simulink subsystem "Drive_Motor"  (R2025b)
settings: Solver=VariableStepAuto  StartTime=0.0  StopTime=10.0  RelTol=1e-3
model mask{channel=0}
  mask prompts: channel "Servo Channel (0-15)"
libraries: raspberrypiCommlib x5
settings Model: Creator=Maken  LastModifiedBy=Maken

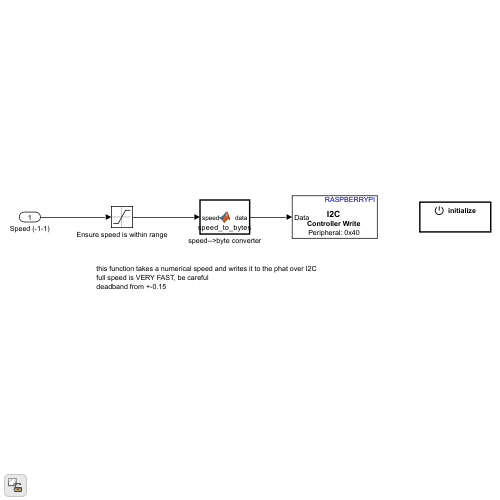
[thumbnail: Simulink's stored preview of the top-level diagram]
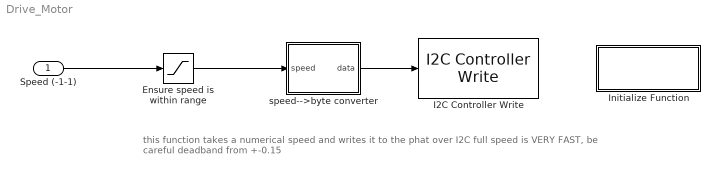
== system Drive_Motor ==
  note: this function takes a numerical speed and writes it to the phat over I2C
      | full speed is VERY FAST, be careful
      | deadband from +-0.15
  Speed (-1-1) : Inport
  Ensure speed is within range : Saturate  UpperLimit=1  LowerLimit=-1
  I2C Controller Write : raspberrypiCommlib/I2C Controller Write  BoardProperty=Pi 5 Model  I2CModule=1  Mode=Master  SlaveAddress=0x40  SlaveByteOrder=LittleEndian  Direction=Transmitter  RegisterAddressMode=on  RegisterAddress=0x06 + (channel * 4)  SlaveDataType=uint8  DataLength=1  NoAck=off  RepeatedStart=off  OutputStatus=off
  Initialize Function : Subsystem  TreatAsAtomicUnit=on
  speed-->byte converter : MATLAB Function  TreatAsAtomicUnit=on
  wires:
  Speed (-1-1)/1 -> Ensure speed is within range/1
  Ensure speed is within range/1 -> speed-->byte converter/1(speed)
  speed-->byte converter/1(data) -> I2C Controller Write/1

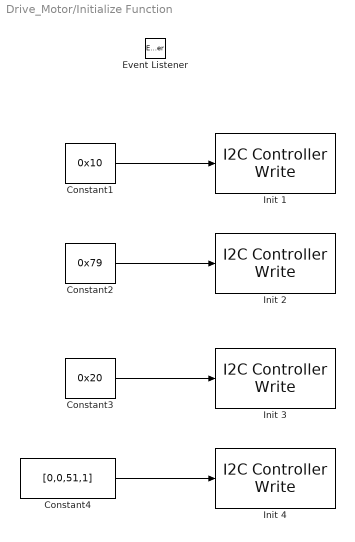
== system Drive_Motor/Initialize Function ==
  Constant1 : Constant  Value=0x10
  Constant2 : Constant  Value=0x79
  Constant3 : Constant  Value=0x20
  Constant4 : Constant  Value=[0,0,51,1]  OutDataTypeStr=uint8
  Event Listener : EventListener  DisableCoverage=on  EventName=reset
  Init 1 : raspberrypiCommlib/I2C Controller Write  BoardProperty=Pi 5 Model  I2CModule=1  Mode=Master  SlaveAddress=0x40  SlaveByteOrder=LittleEndian  Direction=Transmitter  RegisterAddressMode=on  RegisterAddress=0x00  SlaveDataType=uint8  DataLength=1  NoAck=off  RepeatedStart=off  OutputStatus=off
  Init 2 : raspberrypiCommlib/I2C Controller Write  BoardProperty=Pi 5 Model  I2CModule=1  Mode=Master  SlaveAddress=0x40  SlaveByteOrder=LittleEndian  Direction=Transmitter  RegisterAddressMode=on  RegisterAddress=0xFE  SlaveDataType=uint8  DataLength=1  NoAck=off  RepeatedStart=off  OutputStatus=off
  Init 3 : raspberrypiCommlib/I2C Controller Write  BoardProperty=Pi 5 Model  I2CModule=1  Mode=Master  SlaveAddress=0x40  SlaveByteOrder=LittleEndian  Direction=Transmitter  RegisterAddressMode=on  RegisterAddress=0x00  SlaveDataType=uint8  DataLength=1  NoAck=off  RepeatedStart=off  OutputStatus=off
  Init 4 : raspberrypiCommlib/I2C Controller Write  BoardProperty=Pi 5 Model  I2CModule=1  Mode=Master  SlaveAddress=0x40  SlaveByteOrder=LittleEndian  Direction=Transmitter  RegisterAddressMode=on  RegisterAddress=0x06 + (channel * 4)  SlaveDataType=uint8  DataLength=1  NoAck=off  RepeatedStart=off  OutputStatus=off
  wires:
  Constant4/1 -> Init 4/1
  Constant3/1 -> Init 3/1
  Constant2/1 -> Init 2/1
  Constant1/1 -> Init 1/1

== matlab function Drive_Motor/speed-->byte converter ==
  data: speed input; data output
function data = speed_to_bytes(speed)
%#codegen
% speed: -1.0 (full reverse) to +1.0 (full forward), 0 = stop
speed_clamped = max(-1.0, min(1.0, double(speed)));
tick = uint16(round(307 + speed_clamped * 102));
% 307 = neutral, 102 = range to each endpoint (205 ticks total / 2)
off_l = uint8(bitand(tick, uint16(255)));
off_h = uint8(bitshift(tick, -8));
data = [uint8(0), uint8(0), off_l, off_h];
